simulink library "MSP_SP"  (R2016b)
settings: Solver=VariableStepAuto  StartTime=0.0  StopTime=10.0  RelTol=1e-3
undefined symbols (not defined in the file or in its folder): fsw_params
libraries: sensor_processing_libs x2, GPS_processing_lib x1
settings Model: Creator=taylorreynolds  LastModifiedBy=taylorreynolds

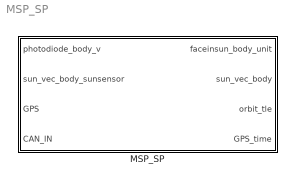
== system MSP_SP ==
  MSP_SP : Subsystem

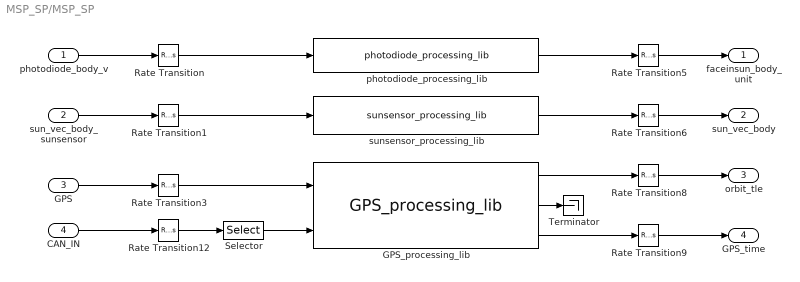
== system MSP_SP/MSP_SP ==
  photodiode_body_v : Inport
  sun_vec_body_sunsensor : Inport  Port=2
  GPS : Inport  Port=3
  CAN_IN : Inport  Port=4
  GPS_processing_lib : GPS_processing_lib/GPS_processing_lib
  Rate Transition : RateTransition  OutPortSampleTime=fsw_params.sensor_processing.MSP_SP.sample_time_s
  Rate Transition1 : RateTransition  OutPortSampleTime=fsw_params.sensor_processing.MSP_SP.sample_time_s
  Rate Transition12 : RateTransition  X0=fsw_params.sensor_processing.gps.JD_J2000_TT  OutPortSampleTime=fsw_params.sensor_processing.MSP_SP.sample_time_s
  Rate Transition3 : RateTransition  X0=fsw_params.sensor_processing.gps.ic.all  OutPortSampleTime=fsw_params.sensor_processing.MSP_SP.sample_time_s
  Rate Transition5 : RateTransition
  Rate Transition6 : RateTransition
  Rate Transition8 : RateTransition  X0=fsw_params.environment.sgp4.orbit_tle
  Rate Transition9 : RateTransition  X0=fsw_params.sensor_processing.gps.ic.time
  Selector : Selector  InputPortWidth=8  IndexOptions=Index vector (dialog)  Indices=8  OutputSizes=1
  Terminator : Terminator
  photodiode_processing_lib : sensor_processing_libs/photodiode_processing_lib
  sunsensor_processing_lib : sensor_processing_libs/sunsensor_processing_lib
  faceinsun_body_unit : Outport
  sun_vec_body : Outport  Port=2
  orbit_tle : Outport  Port=3
  GPS_time : Outport  Port=4
  wires:
  Rate Transition5/1 -> faceinsun_body_unit/1
  photodiode_processing_lib/1 -> Rate Transition5/1
  GPS_processing_lib/3 -> Rate Transition9/1
  GPS_processing_lib/1 -> Rate Transition8/1
  sunsensor_processing_lib/1 -> Rate Transition6/1
  Rate Transition/1 -> photodiode_processing_lib/1
  Rate Transition1/1 -> sunsensor_processing_lib/1
  Rate Transition3/1 -> GPS_processing_lib/1
  GPS_processing_lib/2 -> Terminator/1
  Rate Transition12/1 -> Selector/1
  Selector/1 -> GPS_processing_lib/2
  photodiode_body_v/1 -> Rate Transition/1
  CAN_IN/1 -> Rate Transition12/1
  GPS/1 -> Rate Transition3/1
  sun_vec_body_sunsensor/1 -> Rate Transition1/1
  Rate Transition9/1 -> GPS_time/1
  Rate Transition8/1 -> orbit_tle/1
  Rate Transition6/1 -> sun_vec_body/1
